simulink model "connectwithoutmech_by_indraneel_saki"  (Simulink 10.0)
settings: Solver=ode45  StartTime=0  StopTime=5  MaxStep=5e-4  RelTol=1e-3  EnableMultiTasking=on
libraries: simulink x1
settings Model: Creator=M.Riaz  LastModifiedBy=bhisma  ExtModeTrigMode=oneshot  ExtModeArmWhenConnect=off
settings DataIOCC: SignalLoggingSaveFormat=ModelDataLogs  SaveOutput=off  TimeSaveName=t  SignalLoggingName=sigsOut
settings OptimizationCC: BlockReduction=off  BooleanDataType=off  ExpressionDepthLimit=2147483647  InitFltsAndDblsToZero=on
settings DebuggingCC: SaveWithParameterizedLinksMsg=none  SignalResolutionControl=TryResolveAllWithWarning  MultiTaskDSMMsg=warning  MultiTaskCondExecSysMsg=none  FcnCallInpInsideContextMsg=warning  StateNameClashWarn=warning
settings HardwareCC: TargetUnknown=on
settings GRTTargetCC: GeneratePreprocessorConditionals=Disable all
settings ConfigComp: CovExternalEMLEnable=off

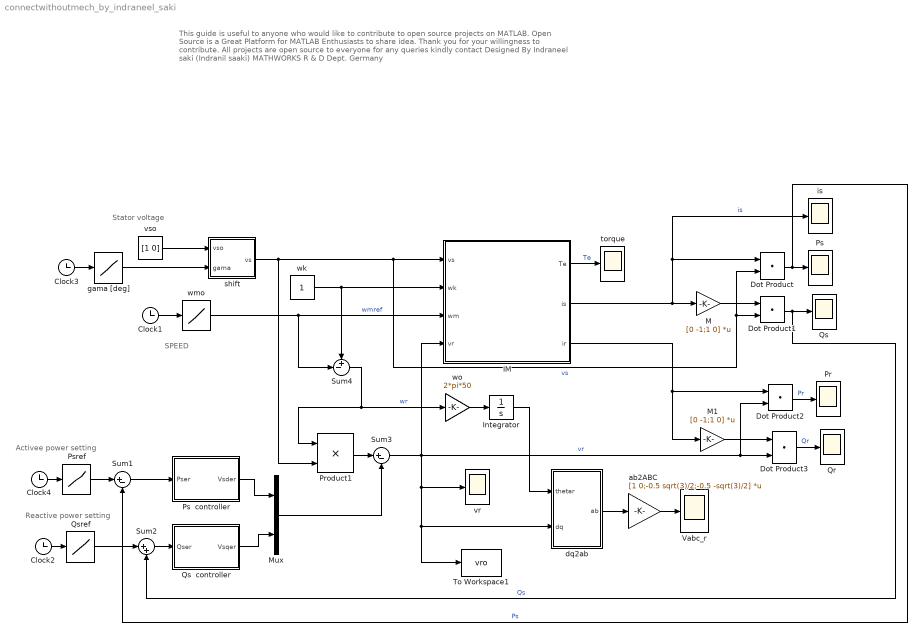
== system connectwithoutmech_by_indraneel_saki ==
  note: SPEED
  note: Reactive power setting
  note: Activee power setting
  note: Stator voltage
  note: This guide is useful to anyone who would like to contribute to open source projects on MATLAB.
      | Open Source is a Great Platform for MATLAB Enthusiasts to share idea. Thank you for your willingness to contribute.
      | All projects are open source to everyone for any queries kindly contact
      | Designed By Indraneel saki (Indranil saaki)
      | MATHWORKS R & D Dept.
      | Germany
  Clock{1..4} (4 alike) : Clock
  Dot Product{,1..3} (4 alike) : DotProduct  InputSameDT=on  OutDataTypeStr=Inherit: Inherit via internal rule
  IM : Subsystem  mask{Rs=0.01, Lsl=0.1, Rr=0.02, Lm=5, Lrl=0.1, wo=2*pi*50}
      mask prompts: Rs "Stator resistance [pu]"; Lsl "Stator leakage inductance [pu]"; Rr "Rotor resistance [pu]"; Lm "Magnetizing inductance [pu]"; Lrl "Rotor leakage inductance [pu]"; wo "base frequency [rad/s]"
      mask Display: disp('DOUBLY-FED\nINDUCTION\nGENERATOR')
  Integrator : Integrator
  M : Gain  Gain=[0 -1;1 0]  Multiplication=Matrix(K*u)  SaturateOnIntegerOverflow=on  OutDataTypeStr=Inherit: Same as input  ParamDataTypeStr=Inherit: Same as input
  M1 : Gain  Gain=[0 -1;1 0]  Multiplication=Matrix(K*u)  SaturateOnIntegerOverflow=on  OutDataTypeStr=Inherit: Same as input  ParamDataTypeStr=Inherit: Same as input
  Mux : Mux  Inputs=2
  Pr : Scope
  Product1 : Product  SaturateOnIntegerOverflow=on  OutDataTypeStr=Inherit: Same as first input
  Ps : Scope
  Ps  controller : Subsystem  mask{Kp=.1, Ki=10, sat=3}
      mask prompts: Kp "Proportional gain (Kp)"; Ki "Integral gain (Ki)"; sat "Saturation limit [pu]"
      mask help: Proportional-Integral Speed Controller
  Psref : Lookup  InputValues=[0 2 2.01 10 ]  Table=[0 0 -1 -1]  SaturateOnIntegerOverflow=on
  Qr : Scope
  Qs : Scope
  Qs  controller : Subsystem  mask{Kp=.1, Ki=10, sat=1000}
      mask prompts: Kp "Proportional gain (Kp)"; Ki "Integral gain (Ki)"; sat "Saturation limit [pu]"
      mask help: Proportional-Integral Speed Controller
  Qsref : Lookup  InputValues=[0 3 3.01 30 ]  Table=[0 0 .5 .5]  SaturateOnIntegerOverflow=on
  Sum1 : Sum  Inputs=|+-  SaturateOnIntegerOverflow=on
  Sum2 : Sum  Inputs=|++  SaturateOnIntegerOverflow=on
  Sum3 : Sum  Inputs=|+-  SaturateOnIntegerOverflow=on
  Sum4 : Sum  Inputs=+-|  SaturateOnIntegerOverflow=on
  To Workspace1 : ToWorkspace  VariableName=vro  SampleTime=-1
  Vabc_r : Scope
  ab2ABC : Gain  Gain=[1 0;-0.5 sqrt(3)/2;-0.5 -sqrt(3)/2]  Multiplication=Matrix(K*u)  SaturateOnIntegerOverflow=on  OutDataTypeStr=Inherit: Same as input  ParamDataTypeStr=Inherit: Same as input
  "dq2ab " : Subsystem
  gama [deg] : Lookup  InputValues="[0  1 1.01 5]"  Table=[0 0 10 10]  SaturateOnIntegerOverflow=on
  is : Scope
  shift : Subsystem
  torque : Scope
  vr : Scope
  vso : Constant  Value=[1 0]
  wk : Constant
  wmo : Lookup  InputValues=[0 4 4.01 20 ]  Table=[.7 .7 1.3 1.3]  SaturateOnIntegerOverflow=on
  wo : Gain  Gain=2*pi*50  SaturateOnIntegerOverflow=on  OutDataTypeStr=Inherit: Same as input  ParamDataTypeStr=Inherit: Same as input
  wires:
  shift/1(vs) -> IM/1(vs), Dot Product/2, Dot Product1/2, Product1/2  "vs"
  wk/1 -> IM/2(wk), Sum4/1
  Dot Product/1 -> Ps/1, Sum1/2  "Ps"
  M/1 -> Dot Product1/1
  Dot Product1/1 -> Qs/1, Sum2/2  "Qs"
  IM/2(is) -> M/1, Dot Product/1, is/1  "is"
  Dot Product2/1 -> Pr/1  "Pr"
  M1/1 -> Dot Product3/1
  Dot Product3/1 -> Qr/1  "Qr"
  IM/3(ir) -> M1/1, Dot Product2/1
  Clock1/1 -> wmo/1
  wmo/1 -> IM/3(wm), Sum4/2  "wmref"
  IM/1(Te) -> torque/1  "Te"
  Qs  controller/1(Vsqer) -> Mux/2
  Sum2/1 -> Qs  controller/1(Qser)
  Sum1/1 -> Ps  controller/1(Pser)
  Ps  controller/1(Vsder) -> Mux/1
  Sum4/1 -> Product1/1, wo/1  "wr"
  Product1/1 -> Sum3/1
  Sum3/1 -> IM/4(vr), Dot Product3/2, Dot Product2/2, vr/1, "dq2ab "/2(dq), To Workspace1/1  "vr"
  Clock4/1 -> Psref/1
  Psref/1 -> Sum1/1
  Clock2/1 -> Qsref/1
  Qsref/1 -> Sum2/1
  Clock3/1 -> gama [deg]/1
  vso/1 -> shift/1(vso)
  gama [deg]/1 -> shift/2(gama)
  "dq2ab "/1(ab) -> ab2ABC/1
  ab2ABC/1 -> Vabc_r/1
  wo/1 -> Integrator/1
  Integrator/1 -> "dq2ab "/1(thetar)
  Mux/1 -> Sum3/2

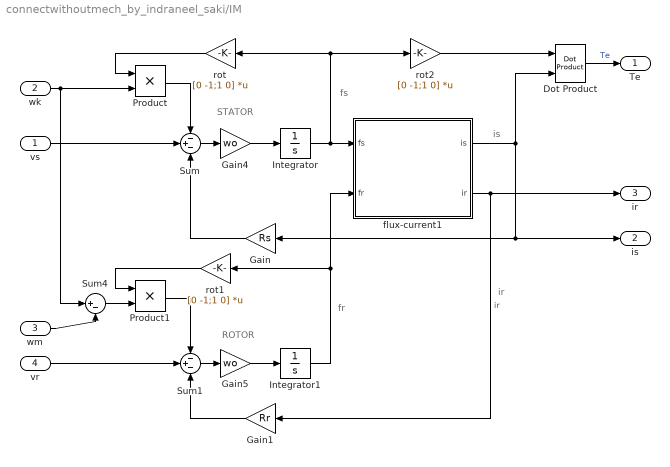
== system connectwithoutmech_by_indraneel_saki/IM ==
  note: fs
  note: fr
  note: is
  note: ir
  note: ROTOR
  note: STATOR
  vs : Inport
  wk : Inport  Port=2
  wm : Inport  Port=3
  vr : Inport  Port=4
  Dot Product : simulink/Math Operations/Dot Product  InputSameDT=on  OutDataType=sfix(16)  OutScaling=2^-10  DoSatur=off
      settings: SourceProductName=Simulink  SourceProductBaseCode=SL
  Gain : Gain  Gain=Rs  SaturateOnIntegerOverflow=on  OutDataTypeStr=Inherit: Same as input  ParamDataTypeStr=Inherit: Same as input
  Gain1 : Gain  Gain=Rr  SaturateOnIntegerOverflow=on  OutDataTypeStr=Inherit: Same as input  ParamDataTypeStr=Inherit: Same as input
  Gain4 : Gain  Gain=wo  SaturateOnIntegerOverflow=on  OutDataTypeStr=Inherit: Same as input  ParamDataTypeStr=Inherit: Same as input
  Gain5 : Gain  Gain=wo  SaturateOnIntegerOverflow=on  OutDataTypeStr=Inherit: Same as input  ParamDataTypeStr=Inherit: Same as input
  Integrator : Integrator  InitialCondition=[0 -1]
  Integrator1 : Integrator  InitialCondition=[0 -1]
  Product : Product  SaturateOnIntegerOverflow=on  InputSameDT=on  OutDataTypeStr=Inherit: Same as first input
  Product1 : Product  SaturateOnIntegerOverflow=on  InputSameDT=on  OutDataTypeStr=Inherit: Same as first input
  Sum : Sum  Inputs=-+-  SaturateOnIntegerOverflow=on  InputSameDT=on  OutDataTypeStr=Inherit: Same as first input
  Sum1 : Sum  Inputs=-+-  SaturateOnIntegerOverflow=on  InputSameDT=on  OutDataTypeStr=Inherit: Same as first input
  Sum4 : Sum  Inputs=|+-  SaturateOnIntegerOverflow=on  InputSameDT=on  OutDataTypeStr=Inherit: Same as first input
  flux-current1 : Subsystem
      mask Display: disp('FLUX-CURRENT\nRELATIONS')
  rot : Gain  Gain=[0 -1;1 0]  Multiplication=Matrix(K*u)  SaturateOnIntegerOverflow=on  OutDataTypeStr=Inherit: Same as input  ParamDataTypeStr=Inherit: Same as input
  rot1 : Gain  Gain=[0 -1;1 0]  Multiplication=Matrix(K*u)  SaturateOnIntegerOverflow=on  OutDataTypeStr=Inherit: Same as input  ParamDataTypeStr=Inherit: Same as input
  rot2 : Gain  Gain=[0 -1;1 0]  Multiplication=Matrix(K*u)  SaturateOnIntegerOverflow=on  OutDataTypeStr=Inherit: Same as input  ParamDataTypeStr=Inherit: Same as input
  Te : Outport
  is : Outport  Port=2
  ir : Outport  Port=3
  wires:
  Gain/1 -> Sum/3
  Gain1/1 -> Sum1/3
  flux-current1/2(ir) -> Gain1/1, ir/1  "ir"
  Integrator/1 -> flux-current1/1(fs), rot/1, rot2/1
  Integrator1/1 -> flux-current1/2(fr), rot1/1
  Product1/1 -> Sum1/1
  rot1/1 -> Product1/1
  Product/1 -> Sum/1
  rot/1 -> Product/1
  rot2/1 -> Dot Product/1
  Sum4/1 -> Product1/2
  Sum/1 -> Gain4/1
  Gain4/1 -> Integrator/1
  Sum1/1 -> Gain5/1
  Gain5/1 -> Integrator1/1
  flux-current1/1(is) -> Gain/1, is/1, Dot Product/2
  Dot Product/1 -> Te/1  "Te"
  vs/1 -> Sum/2
  wk/1 -> Product/2, Sum4/1
  wm/1 -> Sum4/2
  vr/1 -> Sum1/2

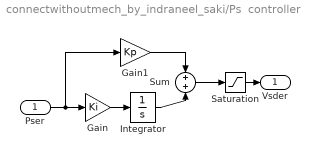
== system connectwithoutmech_by_indraneel_saki/Ps  controller ==
  Pser : Inport
  Gain : Gain  Gain=Ki  SaturateOnIntegerOverflow=on  OutDataTypeStr=Inherit: Same as input  ParamDataTypeStr=Inherit: Same as input
  Gain1 : Gain  Gain=Kp  SaturateOnIntegerOverflow=on  OutDataTypeStr=Inherit: Same as input  ParamDataTypeStr=Inherit: Same as input
  Integrator : Integrator  LimitOutput=on  UpperSaturationLimit=sat  LowerSaturationLimit=-sat
  Saturation : Saturate  UpperLimit=sat  LowerLimit=-sat
  Sum : Sum  SaturateOnIntegerOverflow=on  InputSameDT=on  OutDataTypeStr=Inherit: Same as first input
  Vsder : Outport  InitialOutput=0
  wires:
  Integrator/1 -> Sum/2
  Gain1/1 -> Sum/1
  Gain/1 -> Integrator/1
  Pser/1 -> Gain/1, Gain1/1
  Sum/1 -> Saturation/1
  Saturation/1 -> Vsder/1

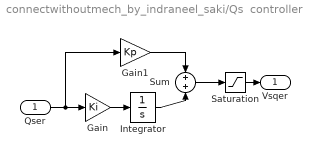
== system connectwithoutmech_by_indraneel_saki/Qs  controller ==
  Qser : Inport
  Gain : Gain  Gain=Ki  SaturateOnIntegerOverflow=on  OutDataTypeStr=Inherit: Same as input  ParamDataTypeStr=Inherit: Same as input
  Gain1 : Gain  Gain=Kp  SaturateOnIntegerOverflow=on  OutDataTypeStr=Inherit: Same as input  ParamDataTypeStr=Inherit: Same as input
  Integrator : Integrator  LimitOutput=on  UpperSaturationLimit=sat  LowerSaturationLimit=-sat
  Saturation : Saturate  UpperLimit=sat  LowerLimit=-sat
  Sum : Sum  SaturateOnIntegerOverflow=on  InputSameDT=on  OutDataTypeStr=Inherit: Same as first input
  Vsqer : Outport  InitialOutput=0
  wires:
  Saturation/1 -> Vsqer/1
  Sum/1 -> Saturation/1
  Qser/1 -> Gain1/1, Gain/1
  Gain/1 -> Integrator/1
  Gain1/1 -> Sum/1
  Integrator/1 -> Sum/2

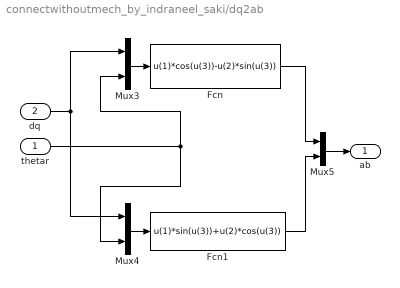
== system connectwithoutmech_by_indraneel_saki/dq2ab  ==
  thetar : Inport
  dq : Inport  Port=2
  Fcn : Fcn  Expr=u(1)*cos(u(3))-u(2)*sin(u(3))
  Fcn1 : Fcn  Expr=u(1)*sin(u(3))+u(2)*cos(u(3))
  Mux3 : Mux  Inputs=2
  Mux4 : Mux  Inputs=2
  Mux5 : Mux  Inputs=2
  ab : Outport
  wires:
  Mux3/1 -> Fcn/1
  Mux4/1 -> Fcn1/1
  dq/1 -> Mux3/1, Mux4/1
  thetar/1 -> Mux3/2, Mux4/2
  Fcn1/1 -> Mux5/2
  Fcn/1 -> Mux5/1
  Mux5/1 -> ab/1

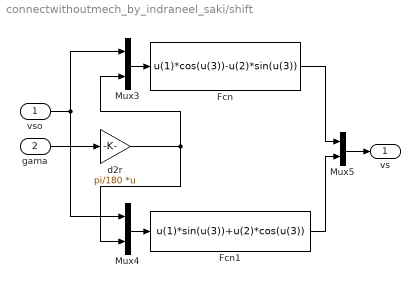
== system connectwithoutmech_by_indraneel_saki/shift ==
  vso : Inport
  gama : Inport  Port=2
  Fcn : Fcn  Expr=u(1)*cos(u(3))-u(2)*sin(u(3))
  Fcn1 : Fcn  Expr=u(1)*sin(u(3))+u(2)*cos(u(3))
  Mux3 : Mux  Inputs=2
  Mux4 : Mux  Inputs=2
  Mux5 : Mux  Inputs=2
  d2r : Gain  Gain=pi/180  Multiplication=Matrix(K*u)  SaturateOnIntegerOverflow=on  OutDataTypeStr=Inherit: Same as input  ParamDataTypeStr=Inherit: Same as input
  vs : Outport
  wires:
  Mux5/1 -> vs/1
  Fcn/1 -> Mux5/1
  Fcn1/1 -> Mux5/2
  gama/1 -> d2r/1
  vso/1 -> Mux4/1, Mux3/1
  Mux4/1 -> Fcn1/1
  Mux3/1 -> Fcn/1
  d2r/1 -> Mux4/2, Mux3/2

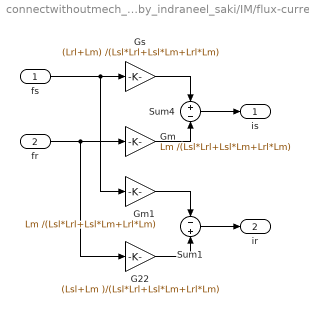
== system connectwithoutmech_by_indraneel_saki/IM/flux-current1 ==
  fs : Inport
  fr : Inport  Port=2
  G22 : Gain  Gain=(Lsl+Lm )/(Lsl*Lrl+Lsl*Lm+Lrl*Lm)  SaturateOnIntegerOverflow=on  OutDataTypeStr=Inherit: Same as input  ParamDataTypeStr=Inherit: Same as input
  Gm : Gain  Gain=Lm /(Lsl*Lrl+Lsl*Lm+Lrl*Lm)  SaturateOnIntegerOverflow=on  OutDataTypeStr=Inherit: Same as input  ParamDataTypeStr=Inherit: Same as input
  Gm1 : Gain  Gain=Lm /(Lsl*Lrl+Lsl*Lm+Lrl*Lm)  SaturateOnIntegerOverflow=on  OutDataTypeStr=Inherit: Same as input  ParamDataTypeStr=Inherit: Same as input
  Gs : Gain  Gain=(Lrl+Lm) /(Lsl*Lrl+Lsl*Lm+Lrl*Lm)  SaturateOnIntegerOverflow=on  OutDataTypeStr=Inherit: Same as input  ParamDataTypeStr=Inherit: Same as input
  Sum1 : Sum  Inputs=-+  SaturateOnIntegerOverflow=on  InputSameDT=on  OutDataTypeStr=Inherit: Same as first input
  Sum4 : Sum  Inputs=+-  SaturateOnIntegerOverflow=on  InputSameDT=on  OutDataTypeStr=Inherit: Same as first input
  is : Outport
  ir : Outport  Port=2
  wires:
  fs/1 -> Gs/1, Gm1/1
  Gs/1 -> Sum4/1
  fr/1 -> Gm/1, G22/1
  Gm/1 -> Sum4/2
  Sum4/1 -> is/1
  Gm1/1 -> Sum1/1
  G22/1 -> Sum1/2
  Sum1/1 -> ir/1
